simulink library "EU_Tapping_Cycle"  (Simulink 7.6)
settings: Solver=ode45  StartTime=0.0  StopTime=10.0  RelTol=1e-3
libraries: carnot x1
settings Model: Creator=lena.frank  LastModifiedBy=drhf

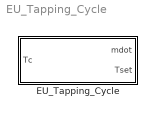
== system EU_Tapping_Cycle ==
  EU_Tapping_Cycle : Subsystem  mask(European tapping cycles){eu_tap=L}
      mask prompts: eu_tap "EU Tapping Cycle Number"
      mask help: European tapping cycles according to EN 13203.
      mask init:
      | % times in h, energies in kWh, massflow in kg/min
      | % will be transformed to s, J at kg/s the end
      | switch(eu_tap)
      |     case 1  % profile 3XS   0.345 kWh
      |         times =    [7.000   7.083   7.250   7.433   7.500   9.000   9.500   11.50   11.75   12.00   12.50   12.75   14.50   15.00   15.50   16.00   18.50   19.00   19.50   21.25   21.50   21.58   21.75 ];
      |         energies = [0.015   0.015   0.015   0.015   0.015   0.015   0.015   0.015   0.015   0.015   0.015   0.015   0.015   0.015   0.015   0.015   0.015   0.015   0.015   0.015   0.015   0.015   0.015 ];
      |         dT_set =   [30      30      30      30      30      30      30      30      30      30      30      30      30      30      30      30      30      30      30      30      30      30      30  ];
      |         mdot =     [2       2       2       2       2       2       2       2       2       2       2       2       2       2       2       2       2       2       2       2       2       2       2   ];
      | 
      |     case 2  % profile XXS   2.1 kWh
      |         times =    [7.000   7.500   8.500   9.500   11.50   11.75   12.00   12.50   12.75   18.00   18.25   18.50   19.00   19.50   20.00   20.75   21.00   21.25   21.58   21.75 ];
      |         energies = [0.105   0.105   0.105   0.105   0.105   0.105   0.105   0.105   0.105   0.105   0.105   0.105   0.105   0.105   0.105   0.105   0.105   0.105   0.105   0.105 ];
      |         dT_set =   [30      30      30      30      30      30      30      30      30      30      30      30      30      30      30      30      30      30      30      30    ];
      |         mdot =     [2       2       2       2       2       2       2       2       2       2       2       2       2       2       2       2       2       2       2       2     ];
      | 
      |     case 3  % profile XS    2.1 kWh
      |         times =    [7.500   12.75   21.50   ];
      |         energies = [0.525   0.525   1.05    ];
      |         dT_set =   [30      30      30      ];
      |         mdot =     [3       3       3       ];
      |     
      |     case 4  % profile S     2.1 kWh
      |         times =    [7.000   7.500   8.500   9.500   11.50   11.75   12.75   18.00   18.25   20.50   21.50   ];
      |         energies = [0.105   0.105   0.105   0.105   0.105   0.105   0.315   0.105   0.105   0.420   0.525   ];
      |         dT_set =   [30      30      30      30      30      30      45      30      30      45      30      ];
      |         mdot =     [3       3       3       3       3       3       4       3       3       4       5       ];
      |     
      |     case 5 % Profile M      5.845 kWh
      |         times =    [7.000 7.083 7.500 8.016 8.250 8.5   8.750 9.000 9.500 10.50 11.50 11.75 12.75 14.50 15.50 16.50 18.00 18.25 18.50 19.00 20.50 21.25 21.5];
      |         energies = [0.105 1.4   0.105 0.105 0.105 0.105 0.105 0.105 0.105 0.105 0.105 0.105 0.315 0.105 0.105 0.105 0.105 0.105 0.105 0.105 0.735 0.105 1.4 ];
      |         dT_set =   [30    30    30    30    30    30    30    30    30    30    30    30    45    30    30    30    30    30    30    30    45    30    30  ];
      |         mdot   =   [3     6     3     3     3     3     3     3     3     3     3     3     4     3     3     3     3     3     3     3     4     3     6   ];
      |         
      |     case 6 % profile L      11.655 kWh
      |         times =    [7.000 7.083 7.500 7.750 8.083 8.416 8.500 8.750 9.000 9.500 10.50 11.50 11.75 12.75 14.50 15.50 16.50 18.00 18.25 18.50 19.00 20.50 21.00 21.5 ];
      |         energies = [0.105 1.4   0.105 0.105 3.605 0.105 0.105 0.105 0.105 0.105 0.105 0.105 0.105 0.315 0.105 0.105 0.105 0.105 0.105 0.105 0.105 0.735 3.605 0.105];
      |         dT_set   = [30    30    30    30    30    30    30    30    30    30    30    30    30    45    30    30    30    30    30    30    30    45    30    30   ];
      |         mdot     = [3     6     3     3     10    3     3     3     3     3     3     3     3     4     3     3     3     3     3     3     3     4     10    3    ];
      |         
      |     case 7  % profile XL      19.07 kWh
      |         times =    [7.000 7.25  7.433 7.75  8.016 8.250 8.500 8.750 9.000 9.500 10.00 10.50 11.00 11.50 11.75 12.75 14.50 15.00 15.50 16.00 16.50 17.00 18.00 18.25 18.50 19.00 20.50 20.76 21.25 21.5 ];
      |         energies = [0.105 1.82  0.105 4.42  0.105 0.105 0.105 0.105 0.105 0.105 0.105 0.105 0.105 0.105 0.105 0.735 0.105 0.105 0.105 0.105 0.105 0.105 0.105 0.105 0.105 0.105 0.735 4.420 0.105 4.42 ];
      |         dT_set   = [30    35    30    30    30    30    30    30    30    30    30    30    30    30    45    45    30    30    30    30    30    30    30    35    35    30    45    35    30    35   ];
      |         mdot     = [3     6     3     10    3     3     3     3     3     3     3     3     3     4     3     3     3     3     3     3     3     4     10    3     3     3     4     10    3     10   ];
      |         
      |     case 8  % profile XXL      24.53 kWh
      |         times =    [7.000 7.25  7.433 7.75  8.016 8.250 8.500 8.750 9.000 9.500 10.00 10.50 11.00 11.50 11.75 12.75 14.50 15.00 15.50 16.00 16.50 17.00 18.00 18.25 18.50 19.00 20.50 20.76 21.25 21.5 ];
      |         energies = [0.105 1.82  0.105 6.24  0.105 0.105 0.105 0.105 0.105 0.105 0.105 0.105 0.105 0.105 0.105 0.735 0.105 0.105 0.105 0.105 0.105 0.105 0.105 0.105 0.105 0.105 0.735 6.240 0.105 6.24 ];
      |         dT_set   = [30    35    30    35    30    30    30    30    30    30    30    35    30    45    45    45    30    30    30    30    30    30    30    35    35    30    45    35    35    35   ];
      |         mdot     = [3     6     3     10    3     3     3     3     3     3     3     3     4     3     3     4     3     3     3     3     3     3     3     3     3     3     4     16    10    16   ];
      |         
      |     case 9  % profile 3XL      46.76 kWh
      |         times =    [7.00  8.016 9.000 10.50 11.75 12.75 15.50 18.50 20.50 21.5 ];
      |         energies = [11.2  5.04  1.68  0.840 1.68  2.520 2.520 3.36  5.88  12.04];
      |         dT_set   = [35    30    30    35    30    45    30    30    45    35   ];
      |         mdot     = [48    24    24    24    24    32    24    24    32    48   ];
      |         
      |     case 10 % profile 4XL      93.52 kWh
      |         times =    [7.000 8.016 9.000 10.50 11.75 12.75 15.50 18.50 20.50 21.5 ];
      |         energies = [22.40 10.08 3.36  1.680 3.360 5.04  5.04  6.72  11.76 24.08];
      |         dT_set   = [35    30    30    30    30    45    30    30    45    35   ];
      |         mdot     = [96    48    48    10    48    64    48    48    64    96   ];
      |         
      |     otherwise
      |         disp('Wrong definition of tapping profile')
      | end
      | energies = energies*36e5;
      | times = times*3600;
      | mdot = mdot/60;
      mask StyleString: popup(3XS|XXS|XS|S|M|L|XL|XXL|3XL|4XL)
      mask Display: disp('EU tapping\n from 3XS\nto 4XL')

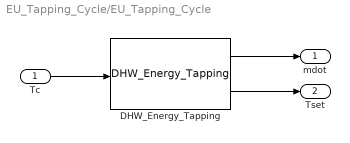
== system EU_Tapping_Cycle/EU_Tapping_Cycle ==
  Tc : Inport
  DHW_Energy_Tapping : carnot/Load/Hot_Water_Tapping/DHW_Energy_Tapping  SystemSampleTime=-1  mdot_nom=1  times=times  energies=energies  dT_set=dT_set  coeffs=mdot
  mdot : Outport
  Tset : Outport  Port=2
  wires:
  DHW_Energy_Tapping/1 -> mdot/1
  DHW_Energy_Tapping/2 -> Tset/1
  Tc/1 -> DHW_Energy_Tapping/1
